simulink model "wss_system_"  (Simulink 7.9)
settings: Solver=FixedStepDiscrete  StartTime=0.0  StopTime=inf  FixedStep=0.05  RelTol=1e-3
undefined symbols (not defined in the file or in its folder): DiscIntNeverNeededParam
libraries: comedi_lib x38, powerlib_extras x19
settings Model: Creator=pppc  LastModifiedBy=pppc  SimulationMode=external  ExtModeTrigDuration=10000  ExtModeAutoUpdateStatusClock=off
settings DataIOCC: MaxDataPoints=10e6
settings OptimizationCC: InitFltsAndDblsToZero=on
settings DebuggingCC: SaveWithParameterizedLinksMsg=none  InheritedTsInSrcMsg=none  StrictBusMsg=Warning
settings RTWCC: SystemTargetFile=lnxxx.tlc  MakeCommand="make_rtw USER_SRCS=\"comedi_lib.c\""  TemplateMakefile=lnxxx_unix.tmf  Description=Linux Near Real-Time Target  ProcessScript=lnxxx_make_rtw_hook  CustomLibrary=/usr/lib/libcomedi.a /usr/lib/x86_64-linux-gnu/libm.a
settings STFCustomTargetCC: CodeReplacementLibrary=ANSI_C  ModelReferenceCompliant=off  GeneratePreprocessorConditionals=Disable all  MatFileLogging=on  SystemTargetFile=lnxxx.tlc
settings CustomProperty: Value=on

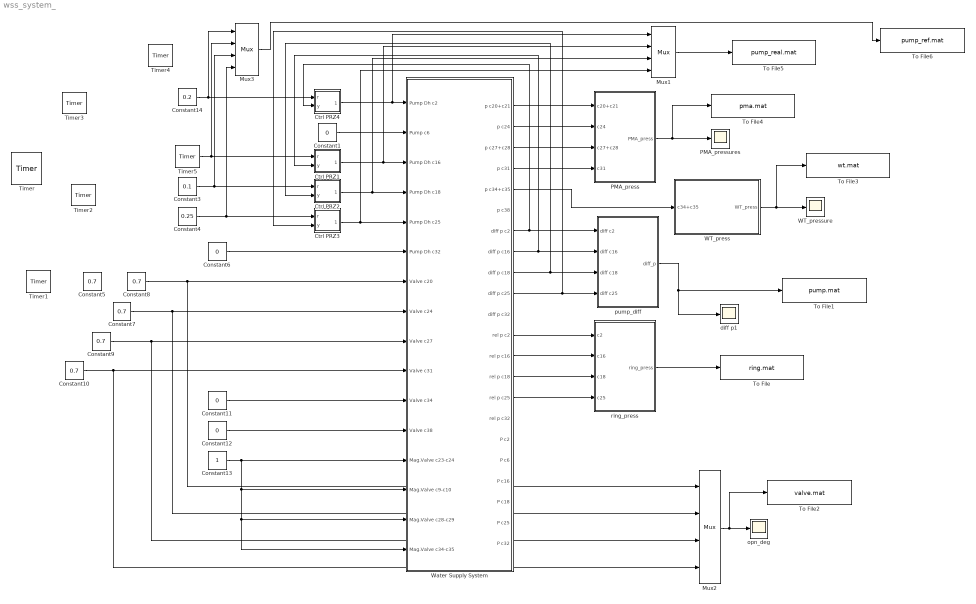
== system wss_system_ ==
  Constant{1,6,11..12} (4 alike) : Constant  Value=0
  Constant{5,7..10} (5 alike) : Constant  Value=0.7
  Constant13 : Constant
  Constant14 : Constant  Value=0.2
  Constant3 : Constant  Value=0.1
  Constant4 : Constant  Value=0.25
  Ctrl PRZ1 : Subsystem
  Ctrl PRZ2 : Subsystem
  Ctrl PRZ3 : Subsystem
  Ctrl PRZ4 : Subsystem
  Mux1 : Mux
  Mux2 : Mux
  Mux3 : Mux
  PMA_press : Subsystem
  PMA_pressures : Scope
      settings: TickLabels=on  ShowLegends=on  TimeRange=500  YMin=0  YMax=0.175  SaveName=Outputs
  Timer : powerlib_extras/Control  Blocks/Timer  t=[0 30 45 60 75 90 105 120 135 150 165]  e=[0.8 1.2 1 2.1 2.8 1.4 2 1.5 1.5 1.5 0.8]
  Timer1 : powerlib_extras/Control  Blocks/Timer  t=[0 300 600 900 1200 1500 1800 2100 2400 2700 3000 3300 3600 3900 4200 4500 4800 5100 5400]  e=[0.7 0.75 0.65 0.7 0.7 0.7 0.7 0.7 0.7 0.7 0.7 0.7 0.7 0.7 0.7 0.7 0.7 0.7 0.7]
  Timer2 : powerlib_extras/Control  Blocks/Timer  t=[0 50 75 100 125 150 175 200 225 250 275 300 325 350 375 400 425 450 475]  e=[0.2 0.22 0.2 0.22 0.18 0.2 0.22 0.18 0.2 0.22 0.18 0.2 0.22 0.18 0.2 0.2 0.22 0.18 0.2]
  Timer3 : powerlib_extras/Control  Blocks/Timer  t=[0 120 240 360 480 600 720 840 960 1080 1200 1320 1440 1560 1680 1800 1920 2040 2160]  e=[0.2 0.215 0.19 0.2 0.215 0.19 0.2 0.215 0.19 0.2 0.215 0.19 0.2 0.215 0.19 0.2 0.2 0.2 0.2]
  Timer4 : powerlib_extras/Control  Blocks/Timer  t=[0 1800 3600]  e=[0.2 0.19 0.2]
  Timer5 : powerlib_extras/Control  Blocks/Timer  t=[0 1800 3600 12600 14400]  e=[0.2 0.213 0.2 0.18 0.2]
  To File : ToFile  Filename=ring.mat  MatrixName=ring_pressure
  To File1 : ToFile  Filename=pump.mat  MatrixName=pump_pressure
  To File2 : ToFile  Filename=valve.mat  MatrixName=valve_OD
  To File3 : ToFile  Filename=wt.mat  MatrixName=wt_pressure
  To File4 : ToFile  Filename=pma.mat  MatrixName=pma_pressure
  To File5 : ToFile  Filename=pump_real.mat  MatrixName=pump_pressure_r  SampleTime=0.05
  To File6 : ToFile  Filename=pump_ref.mat  MatrixName=pump_pressure_ref  SampleTime=0.05
  WT_press : Subsystem
  WT_pressure : Scope
      settings: TickLabels=on  ShowLegends=on  TimeRange=500  YMin=0.124  YMax=0.1245  SaveName=Outputs4
  Water Supply System : Subsystem
  diff p1 : Scope
      settings: TickLabels=on  ShowLegends=on  TimeRange=500  YMin=-0.025  YMax=0.275  SaveName=Outputs5
  opn_deg : Scope
      settings: TickLabels=on  ShowLegends=on  TimeRange=500  YMin=0.699  YMax=0.72  SaveName=Outputs3
  pump_diff : Subsystem
  ring_press : Subsystem
  wires:
  Constant1/1 -> Water Supply System/2(Pump c6)
  Constant11/1 -> Water Supply System/11(Valve c34)
  Constant12/1 -> Water Supply System/12(Valve c38)
  Constant6/1 -> Water Supply System/6(Pump Dh c32)
  Constant13/1 -> Water Supply System/13(Mag.Valve c23-c24), Water Supply System/14(Mag.Valve c9-c10), Water Supply System/15(Mag.Valve c28-c29), Water Supply System/16(Mag.Valve c34-c35)
  Water Supply System/1(p c20+c21) -> PMA_press/1(c20+c21)
  Water Supply System/2(p c24) -> PMA_press/2(c24)
  Water Supply System/3(p c27+c28) -> PMA_press/3(c27+c28)
  Water Supply System/4(p c31) -> PMA_press/4(c31)
  PMA_press/1(PMA_press) -> PMA_pressures/1, To File4/1
  ring_press/1(ring_press) -> To File/1
  Water Supply System/7(diff p c2) -> pump_diff/1(diff c2), Ctrl PRZ4/2(y)
  Water Supply System/8(diff p c16) -> pump_diff/2(diff c16), Ctrl PRZ1/2(y)
  Water Supply System/10(diff p c25) -> pump_diff/4(diff c25), Ctrl PRZ3/2(y)
  Water Supply System/12(rel p c2) -> ring_press/1(c2)
  Water Supply System/13(rel p c16) -> ring_press/2(c16)
  Water Supply System/14(rel p c18) -> ring_press/3(c18)
  Water Supply System/15(rel p c25) -> ring_press/4(c25)
  Water Supply System/9(diff p c18) -> pump_diff/3(diff c18), Ctrl PRZ2/2(y)
  Mux2/1 -> opn_deg/1, To File2/1
  Constant8/1 -> Water Supply System/7(Valve c20), Mux2/1
  Constant7/1 -> Water Supply System/8(Valve c24), Mux2/2
  Constant9/1 -> Water Supply System/9(Valve c27), Mux2/3
  Constant10/1 -> Water Supply System/10(Valve c31), Mux2/4
  Water Supply System/5(p c34+c35) -> WT_press/1(c34+c35)
  WT_press/1(WT_press) -> WT_pressure/1, To File3/1
  pump_diff/1(diff_p) -> diff p1/1, To File1/1
  Ctrl PRZ3/1(Out1) -> Water Supply System/5(Pump Dh c25), Mux1/4
  Ctrl PRZ2/1(Out1) -> Water Supply System/4(Pump Dh c18), Mux1/3
  Ctrl PRZ1/1(Out1) -> Water Supply System/3(Pump Dh c16), Mux1/2
  Constant3/1 -> Ctrl PRZ2/1(r), Mux3/3
  Constant4/1 -> Ctrl PRZ3/1(r), Mux3/4
  Ctrl PRZ4/1(Out1) -> Water Supply System/1(Pump Dh c2), Mux1/1
  Timer5/1 -> Ctrl PRZ1/1(r), Mux3/2
  Constant14/1 -> Ctrl PRZ4/1(r), Mux3/1
  Mux1/1 -> To File5/1
  Mux3/1 -> To File6/1

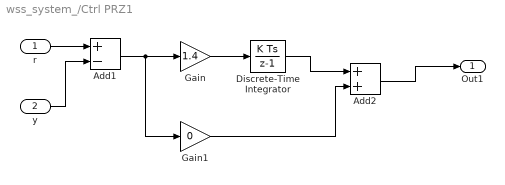
== system wss_system_/Ctrl PRZ1 ==
  r : Inport
  y : Inport  Port=2
  Add1 : Sum  Inputs=+-
  Add2 : Sum
  Discrete-Time Integrator : DiscreteIntegrator  SampleTime=0.05  ICPrevOutput=DiscIntNeverNeededParam  ICPrevScaledInput=DiscIntNeverNeededParam
  Gain : Gain  Gain=1.4
  Gain1 : Gain  Gain=0
  Out1 : Outport
  wires:
  Add2/1 -> Out1/1
  Gain1/1 -> Add2/2
  Discrete-Time Integrator/1 -> Add2/1
  r/1 -> Add1/1
  y/1 -> Add1/2
  Add1/1 -> Gain1/1, Gain/1
  Gain/1 -> Discrete-Time Integrator/1

== system wss_system_/Ctrl PRZ2 ==
  r : Inport
  y : Inport  Port=2
  Add1 : Sum  Inputs=+-
  Add2 : Sum
  Discrete-Time Integrator : DiscreteIntegrator  SampleTime=0.05  ICPrevOutput=DiscIntNeverNeededParam  ICPrevScaledInput=DiscIntNeverNeededParam
  Gain : Gain  Gain=1.6
  Gain1 : Gain  Gain=0
  Out1 : Outport
  wires:
  Gain/1 -> Discrete-Time Integrator/1
  Add1/1 -> Gain/1, Gain1/1
  y/1 -> Add1/2
  r/1 -> Add1/1
  Gain1/1 -> Add2/2
  Discrete-Time Integrator/1 -> Add2/1
  Add2/1 -> Out1/1

== system wss_system_/Ctrl PRZ3 ==
  r : Inport
  y : Inport  Port=2
  Add1 : Sum  Inputs=+-
  Add2 : Sum
  Discrete-Time Integrator : DiscreteIntegrator  SampleTime=0.05  ICPrevOutput=DiscIntNeverNeededParam  ICPrevScaledInput=DiscIntNeverNeededParam
  Gain : Gain  Gain=1.4
  Gain1 : Gain  Gain=0
  Out1 : Outport
  wires:
  r/1 -> Add1/1
  y/1 -> Add1/2
  Add1/1 -> Gain/1, Gain1/1
  Gain/1 -> Discrete-Time Integrator/1
  Add2/1 -> Out1/1
  Discrete-Time Integrator/1 -> Add2/1
  Gain1/1 -> Add2/2

== system wss_system_/Ctrl PRZ4 ==
  r : Inport
  y : Inport  Port=2
  Add1 : Sum  Inputs=+-
  Add2 : Sum
  Discrete-Time Integrator : DiscreteIntegrator  SampleTime=0.05  ICPrevOutput=DiscIntNeverNeededParam  ICPrevScaledInput=DiscIntNeverNeededParam
  Gain : Gain  Gain=1.4
  Gain1 : Gain  Gain=0
  Out1 : Outport
  wires:
  Gain/1 -> Discrete-Time Integrator/1
  Add1/1 -> Gain/1, Gain1/1
  y/1 -> Add1/2
  r/1 -> Add1/1
  Discrete-Time Integrator/1 -> Add2/1
  Gain1/1 -> Add2/2
  Add2/1 -> Out1/1

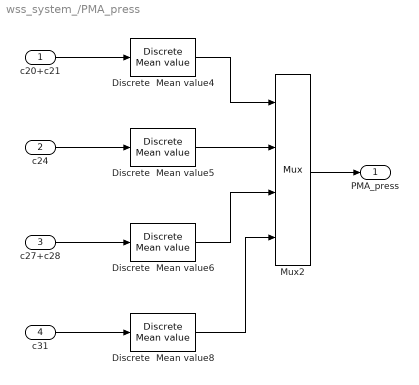
== system wss_system_/PMA_press ==
  c20+c21 : Inport
  c24 : Inport  Port=2
  c27+c28 : Inport  Port=3
  c31 : Inport  Port=4
  Discrete  Mean value{4..6,8} (4 alike) : powerlib_extras/Discrete Measurements/Discrete  Mean value  Freq=0.2  Vinit=0  Ts=0.05
  Mux2 : Mux
  PMA_press : Outport
  wires:
  c20+c21/1 -> Discrete  Mean value4/1
  c27+c28/1 -> Discrete  Mean value6/1
  c24/1 -> Discrete  Mean value5/1
  c31/1 -> Discrete  Mean value8/1
  Mux2/1 -> PMA_press/1
  Discrete  Mean value4/1 -> Mux2/1
  Discrete  Mean value5/1 -> Mux2/2
  Discrete  Mean value6/1 -> Mux2/3
  Discrete  Mean value8/1 -> Mux2/4

== system wss_system_/WT_press ==
  c34+c35 : Inport
  Discrete  Mean value4 : powerlib_extras/Discrete Measurements/Discrete  Mean value  Freq=0.2  Vinit=0  Ts=0.05
  WT_press : Outport
  wires:
  Discrete  Mean value4/1 -> WT_press/1
  c34+c35/1 -> Discrete  Mean value4/1

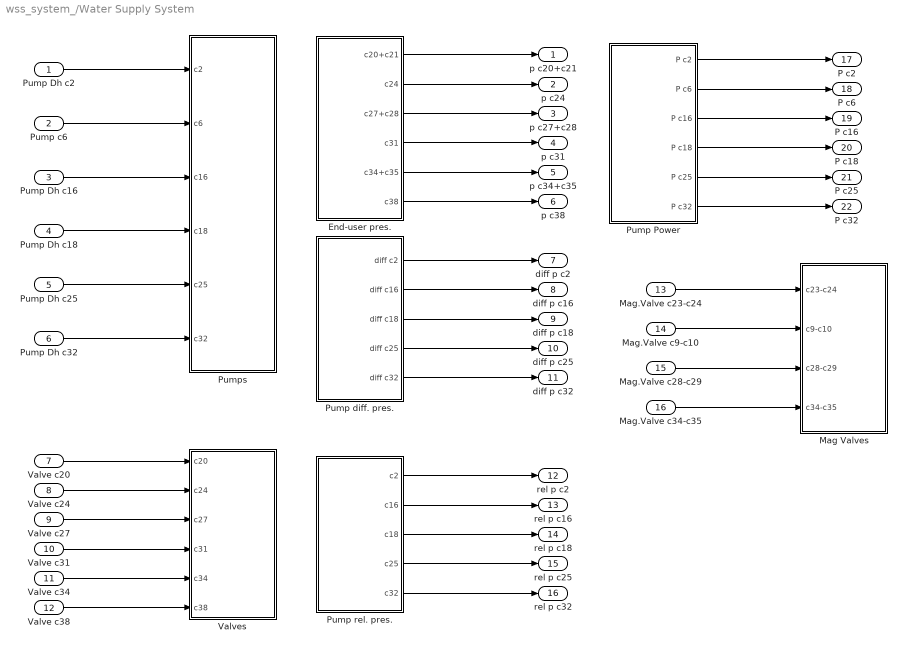
== system wss_system_/Water Supply System ==
  Pump Dh c2 : Inport
  Pump c6 : Inport  Port=2
  Pump Dh c16 : Inport  Port=3
  Pump Dh c18 : Inport  Port=4
  Pump Dh c25 : Inport  Port=5
  Pump Dh c32 : Inport  Port=6
  Valve c20 : Inport  Port=7
  Valve c24 : Inport  Port=8
  Valve c27 : Inport  Port=9
  Valve c31 : Inport  Port=10
  Valve c34 : Inport  Port=11
  Valve c38 : Inport  Port=12
  Mag.Valve c23-c24 : Inport  Port=13
  Mag.Valve c9-c10 : Inport  Port=14
  Mag.Valve c28-c29 : Inport  Port=15
  Mag.Valve c34-c35 : Inport  Port=16
  End-user pres. : Subsystem
  Mag Valves : Subsystem
  Pump Power : Subsystem
  Pump diff. pres. : Subsystem
  Pump rel. pres. : Subsystem
  Pumps : Subsystem
  Valves : Subsystem
  p c20+c21 : Outport
  p c24 : Outport  Port=2
  p c27+c28 : Outport  Port=3
  p c31 : Outport  Port=4
  p c34+c35 : Outport  Port=5
  p c38 : Outport  Port=6
  diff p c2 : Outport  Port=7
  diff p c16 : Outport  Port=8
  diff p c18 : Outport  Port=9
  diff p c25 : Outport  Port=10
  diff p c32 : Outport  Port=11
  rel p c2 : Outport  Port=12
  rel p c16 : Outport  Port=13
  rel p c18 : Outport  Port=14
  rel p c25 : Outport  Port=15
  rel p c32 : Outport  Port=16
  P c2 : Outport  Port=17
  P c6 : Outport  Port=18
  P c16 : Outport  Port=19
  P c18 : Outport  Port=20
  P c25 : Outport  Port=21
  P c32 : Outport  Port=22
  wires:
  Pump diff. pres./1(diff c2) -> diff p c2/1
  Valve c20/1 -> Valves/1(c20)
  Valve c24/1 -> Valves/2(c24)
  Valve c27/1 -> Valves/3(c27)
  Valve c31/1 -> Valves/4(c31)
  Valve c34/1 -> Valves/5(c34)
  Valve c38/1 -> Valves/6(c38)
  Pump rel. pres./1(c2) -> rel p c2/1
  Pump rel. pres./3(c18) -> rel p c18/1
  Pump rel. pres./4(c25) -> rel p c25/1
  Pump diff. pres./3(diff c18) -> diff p c18/1
  End-user pres./3(c27+c28) -> p c27+c28/1
  End-user pres./4(c31) -> p c31/1
  End-user pres./6(c38) -> p c38/1
  Pump rel. pres./5(c32) -> rel p c32/1
  Pump rel. pres./2(c16) -> rel p c16/1
  End-user pres./5(c34+c35) -> p c34+c35/1
  End-user pres./1(c20+c21) -> p c20+c21/1
  End-user pres./2(c24) -> p c24/1
  Pump diff. pres./5(diff c32) -> diff p c32/1
  Pump diff. pres./4(diff c25) -> diff p c25/1
  Pump diff. pres./2(diff c16) -> diff p c16/1
  Pump Dh c2/1 -> Pumps/1(c2)
  Pump c6/1 -> Pumps/2(c6)
  Pump Dh c16/1 -> Pumps/3(c16)
  Pump Dh c18/1 -> Pumps/4(c18)
  Pump Dh c25/1 -> Pumps/5(c25)
  Pump Dh c32/1 -> Pumps/6(c32)
  Pump Power/1(P c2) -> P c2/1
  Pump Power/2(P c6) -> P c6/1
  Pump Power/3(P c16) -> P c16/1
  Pump Power/4(P c18) -> P c18/1
  Pump Power/5(P c25) -> P c25/1
  Pump Power/6(P c32) -> P c32/1
  Mag.Valve c23-c24/1 -> Mag Valves/1(c23-c24)
  Mag.Valve c9-c10/1 -> Mag Valves/2(c9-c10)
  Mag.Valve c28-c29/1 -> Mag Valves/3(c28-c29)
  Mag.Valve c34-c35/1 -> Mag Valves/4(c34-c35)

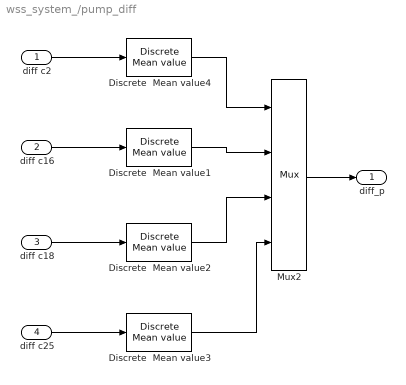
== system wss_system_/pump_diff ==
  diff c2 : Inport
  diff c16 : Inport  Port=2
  diff c18 : Inport  Port=3
  diff c25 : Inport  Port=4
  Discrete  Mean value{1..4} (4 alike) : powerlib_extras/Discrete Measurements/Discrete  Mean value  Freq=0.2  Vinit=0  Ts=0.05
  Mux2 : Mux
  diff_p : Outport
  wires:
  Discrete  Mean value3/1 -> Mux2/4
  Discrete  Mean value2/1 -> Mux2/3
  Discrete  Mean value1/1 -> Mux2/2
  Discrete  Mean value4/1 -> Mux2/1
  Mux2/1 -> diff_p/1
  diff c25/1 -> Discrete  Mean value3/1
  diff c16/1 -> Discrete  Mean value1/1
  diff c18/1 -> Discrete  Mean value2/1
  diff c2/1 -> Discrete  Mean value4/1

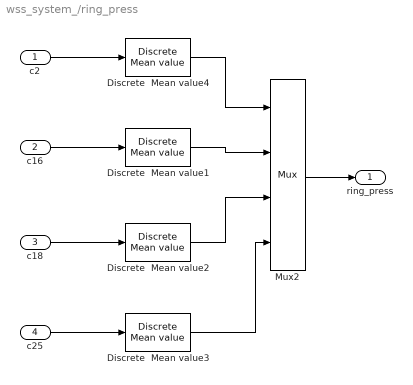
== system wss_system_/ring_press ==
  c2 : Inport
  c16 : Inport  Port=2
  c18 : Inport  Port=3
  c25 : Inport  Port=4
  Discrete  Mean value{1..4} (4 alike) : powerlib_extras/Discrete Measurements/Discrete  Mean value  Freq=0.2  Vinit=0  Ts=0.05
  Mux2 : Mux
  ring_press : Outport
  wires:
  c2/1 -> Discrete  Mean value4/1
  c18/1 -> Discrete  Mean value2/1
  c16/1 -> Discrete  Mean value1/1
  c25/1 -> Discrete  Mean value3/1
  Mux2/1 -> ring_press/1
  Discrete  Mean value4/1 -> Mux2/1
  Discrete  Mean value1/1 -> Mux2/2
  Discrete  Mean value2/1 -> Mux2/3
  Discrete  Mean value3/1 -> Mux2/4

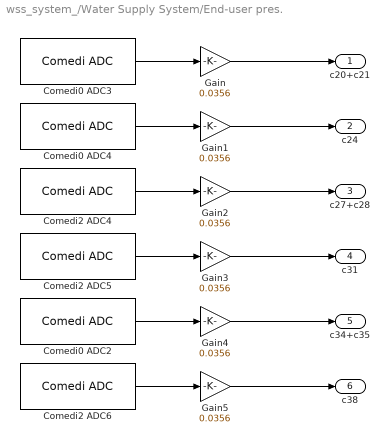
== system wss_system_/Water Supply System/End-user pres. ==
  Comedi0 ADC2 : comedi_lib/Comedi ADC  dev=comedi0  chan=2  range=0  aref=ground  dt=-1
  Comedi0 ADC3 : comedi_lib/Comedi ADC  dev=comedi0  chan=3  range=0  aref=ground  dt=-1
  Comedi0 ADC4 : comedi_lib/Comedi ADC  dev=comedi0  chan=4  range=0  aref=ground  dt=-1
  Comedi2 ADC4 : comedi_lib/Comedi ADC  dev=comedi2  chan=4  range=0  aref=ground  dt=-1
  Comedi2 ADC5 : comedi_lib/Comedi ADC  dev=comedi2  chan=5  range=0  aref=ground  dt=-1
  Comedi2 ADC6 : comedi_lib/Comedi ADC  dev=comedi2  chan=6  range=0  aref=ground  dt=-1
  Gain{,1..5} (6 alike) : Gain  Gain=0.0356
  c20+c21 : Outport
  c24 : Outport  Port=2
  c27+c28 : Outport  Port=3
  c31 : Outport  Port=4
  c34+c35 : Outport  Port=5
  c38 : Outport  Port=6
  wires:
  Comedi0 ADC3/1 -> Gain/1
  Gain/1 -> c20+c21/1
  Comedi0 ADC4/1 -> Gain1/1
  Gain1/1 -> c24/1
  Comedi2 ADC4/1 -> Gain2/1
  Gain2/1 -> c27+c28/1
  Comedi2 ADC5/1 -> Gain3/1
  Gain3/1 -> c31/1
  Comedi0 ADC2/1 -> Gain4/1
  Gain4/1 -> c34+c35/1
  Comedi2 ADC6/1 -> Gain5/1
  Gain5/1 -> c38/1

== system wss_system_/Water Supply System/Mag Valves ==
  c23-c24 : Inport
  c9-c10 : Inport  Port=2
  c28-c29 : Inport  Port=3
  c34-c35 : Inport  Port=4
  Comedi0 DO0 : comedi_lib/Comedi DO  dev=comedi0  chan=0  threshold=0.5
  Comedi0 DO1 : comedi_lib/Comedi DO  dev=comedi0  chan=1  threshold=0.5
  Comedi0 DO2 : comedi_lib/Comedi DO  dev=comedi0  chan=2  threshold=0.5
  Comedi0 DO3 : comedi_lib/Comedi DO  dev=comedi0  chan=3  threshold=0.5
  wires:
  c23-c24/1 -> Comedi0 DO0/1
  c9-c10/1 -> Comedi0 DO1/1
  c28-c29/1 -> Comedi0 DO2/1
  c34-c35/1 -> Comedi0 DO3/1

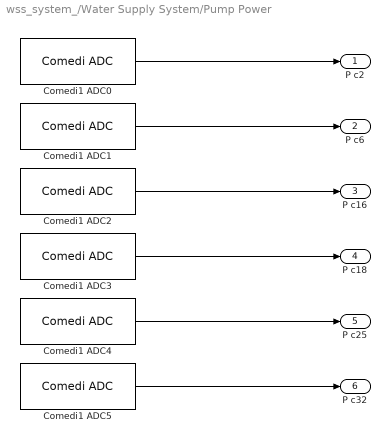
== system wss_system_/Water Supply System/Pump Power ==
  Comedi1 ADC0 : comedi_lib/Comedi ADC  dev=comedi1  chan=0  range=0  aref=ground  dt=-1
  Comedi1 ADC1 : comedi_lib/Comedi ADC  dev=comedi1  chan=1  range=0  aref=ground  dt=-1
  Comedi1 ADC2 : comedi_lib/Comedi ADC  dev=comedi1  chan=2  range=0  aref=ground  dt=-1
  Comedi1 ADC3 : comedi_lib/Comedi ADC  dev=comedi1  chan=3  range=0  aref=ground  dt=-1
  Comedi1 ADC4 : comedi_lib/Comedi ADC  dev=comedi1  chan=4  range=0  aref=ground  dt=-1
  Comedi1 ADC5 : comedi_lib/Comedi ADC  dev=comedi1  chan=5  range=0  aref=ground  dt=-1
  P c2 : Outport
  P c6 : Outport  Port=2
  P c16 : Outport  Port=3
  P c18 : Outport  Port=4
  P c25 : Outport  Port=5
  P c32 : Outport  Port=6
  wires:
  Comedi1 ADC5/1 -> P c32/1
  Comedi1 ADC1/1 -> P c6/1
  Comedi1 ADC3/1 -> P c18/1
  Comedi1 ADC4/1 -> P c25/1
  Comedi1 ADC2/1 -> P c16/1
  Comedi1 ADC0/1 -> P c2/1

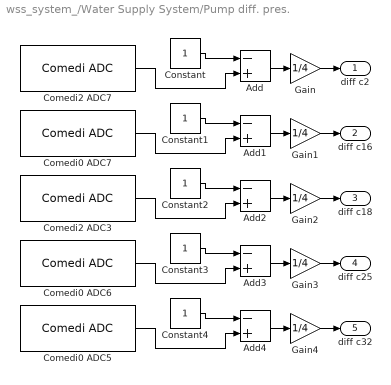
== system wss_system_/Water Supply System/Pump diff. pres. ==
  Add{,1..4} (5 alike) : Sum  Inputs=-+
  Comedi0 ADC5 : comedi_lib/Comedi ADC  dev=comedi0  chan=5  range=0  aref=ground  dt=-1
  Comedi0 ADC6 : comedi_lib/Comedi ADC  dev=comedi0  chan=6  range=0  aref=ground  dt=-1
  Comedi0 ADC7 : comedi_lib/Comedi ADC  dev=comedi0  chan=7  range=0  aref=ground  dt=-1
  Comedi2 ADC3 : comedi_lib/Comedi ADC  dev=comedi2  chan=3  range=0  aref=ground  dt=-1
  Comedi2 ADC7 : comedi_lib/Comedi ADC  dev=comedi2  chan=7  range=0  aref=ground  dt=-1
  Constant{,1..4} (5 alike) : Constant
  Gain{,1..4} (5 alike) : Gain  Gain=1/4
  diff c2 : Outport
  diff c16 : Outport  Port=2
  diff c18 : Outport  Port=3
  diff c25 : Outport  Port=4
  diff c32 : Outport  Port=5
  wires:
  Constant/1 -> Add/1
  Add/1 -> Gain/1
  Gain/1 -> diff c2/1
  Constant1/1 -> Add1/1
  Add1/1 -> Gain1/1
  Constant2/1 -> Add2/1
  Add2/1 -> Gain2/1
  Constant3/1 -> Add3/1
  Add3/1 -> Gain3/1
  Constant4/1 -> Add4/1
  Add4/1 -> Gain4/1
  Comedi2 ADC7/1 -> Add/2
  Comedi0 ADC7/1 -> Add1/2
  Comedi2 ADC3/1 -> Add2/2
  Comedi0 ADC6/1 -> Add3/2
  Comedi0 ADC5/1 -> Add4/2
  Gain1/1 -> diff c16/1
  Gain2/1 -> diff c18/1
  Gain3/1 -> diff c25/1
  Gain4/1 -> diff c32/1

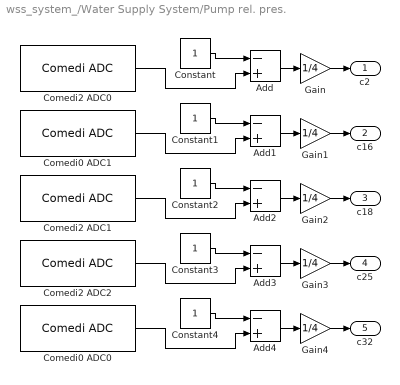
== system wss_system_/Water Supply System/Pump rel. pres. ==
  Add{,1..4} (5 alike) : Sum  Inputs=-+
  Comedi0 ADC0 : comedi_lib/Comedi ADC  dev=comedi0  chan=0  range=0  aref=ground  dt=-1
  Comedi0 ADC1 : comedi_lib/Comedi ADC  dev=comedi0  chan=1  range=0  aref=ground  dt=-1
  Comedi2 ADC0 : comedi_lib/Comedi ADC  dev=comedi2  chan=0  range=0  aref=ground  dt=-1
  Comedi2 ADC1 : comedi_lib/Comedi ADC  dev=comedi2  chan=1  range=0  aref=ground  dt=-1
  Comedi2 ADC2 : comedi_lib/Comedi ADC  dev=comedi2  chan=2  range=0  aref=ground  dt=-1
  Constant{,1..4} (5 alike) : Constant
  Gain{,1..4} (5 alike) : Gain  Gain=1/4
  c2 : Outport
  c16 : Outport  Port=2
  c18 : Outport  Port=3
  c25 : Outport  Port=4
  c32 : Outport  Port=5
  wires:
  Constant/1 -> Add/1
  Add/1 -> Gain/1
  Comedi2 ADC0/1 -> Add/2
  Gain/1 -> c2/1
  Constant1/1 -> Add1/1
  Add1/1 -> Gain1/1
  Constant2/1 -> Add2/1
  Add2/1 -> Gain2/1
  Constant3/1 -> Add3/1
  Add3/1 -> Gain3/1
  Constant4/1 -> Add4/1
  Add4/1 -> Gain4/1
  Comedi0 ADC1/1 -> Add1/2
  Gain1/1 -> c16/1
  Comedi2 ADC1/1 -> Add2/2
  Gain2/1 -> c18/1
  Comedi2 ADC2/1 -> Add3/2
  Gain3/1 -> c25/1
  Comedi0 ADC0/1 -> Add4/2
  Gain4/1 -> c32/1

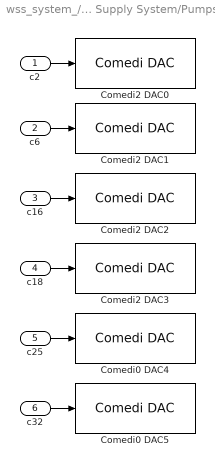
== system wss_system_/Water Supply System/Pumps ==
  c2 : Inport
  c6 : Inport  Port=2
  c16 : Inport  Port=3
  c18 : Inport  Port=4
  c25 : Inport  Port=5
  c32 : Inport  Port=6
  Comedi0 DAC4 : comedi_lib/Comedi DAC  dev=comedi0  chan=4  range=0  aref=ground
  Comedi0 DAC5 : comedi_lib/Comedi DAC  dev=comedi0  chan=5  range=0  aref=ground
  Comedi2 DAC0 : comedi_lib/Comedi DAC  dev=comedi2  chan=0  range=0  aref=ground
  Comedi2 DAC1 : comedi_lib/Comedi DAC  dev=comedi2  chan=1  range=0  aref=ground
  Comedi2 DAC2 : comedi_lib/Comedi DAC  dev=comedi2  chan=2  range=0  aref=ground
  Comedi2 DAC3 : comedi_lib/Comedi DAC  dev=comedi2  chan=3  range=0  aref=ground
  wires:
  c2/1 -> Comedi2 DAC0/1
  c6/1 -> Comedi2 DAC1/1
  c16/1 -> Comedi2 DAC2/1
  c18/1 -> Comedi2 DAC3/1
  c25/1 -> Comedi0 DAC4/1
  c32/1 -> Comedi0 DAC5/1

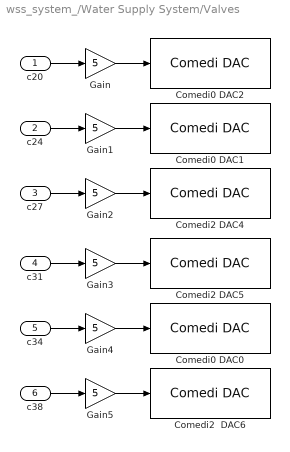
== system wss_system_/Water Supply System/Valves ==
  c20 : Inport
  c24 : Inport  Port=2
  c27 : Inport  Port=3
  c31 : Inport  Port=4
  c34 : Inport  Port=5
  c38 : Inport  Port=6
  Comedi0 DAC0 : comedi_lib/Comedi DAC  dev=comedi0  chan=0  range=0  aref=ground
  Comedi0 DAC1 : comedi_lib/Comedi DAC  dev=comedi0  chan=1  range=0  aref=ground
  Comedi0 DAC2 : comedi_lib/Comedi DAC  dev=comedi0  chan=2  range=0  aref=ground
  Comedi2  DAC6 : comedi_lib/Comedi DAC  dev=comedi2  chan=6  range=0  aref=ground
  Comedi2 DAC4 : comedi_lib/Comedi DAC  dev=comedi2  chan=4  range=0  aref=ground
  Comedi2 DAC5 : comedi_lib/Comedi DAC  dev=comedi2  chan=5  range=0  aref=ground
  Gain{,1..5} (6 alike) : Gain  Gain=5
  wires:
  c20/1 -> Gain/1
  Gain/1 -> Comedi0 DAC2/1
  c24/1 -> Gain1/1
  Gain1/1 -> Comedi0 DAC1/1
  c27/1 -> Gain2/1
  Gain2/1 -> Comedi2 DAC4/1
  c31/1 -> Gain3/1
  Gain3/1 -> Comedi2 DAC5/1
  c34/1 -> Gain4/1
  Gain4/1 -> Comedi0 DAC0/1
  c38/1 -> Gain5/1
  Gain5/1 -> Comedi2  DAC6/1
